simulink library "Soft_Starter_PLL"  (R2024a)
settings: Solver=VariableStepAuto  StartTime=0.0  StopTime=10.0  RelTol=1e-3
undefined symbols (not defined in the file or in its folder): D1, lagging, pulse
libraries: spsThyristorLib x6, spsThreePhaseParallelRLCBranchLib x3, spsThreePhaseBreakerLib x3, spsPLL3phLib x1, spsPulseGeneratorThyristor6PulseLib x1, simulink x1, spsThreePhaseVIMeasurementLib x1
settings Model: Creator=gshma  LastModifiedBy=gshma

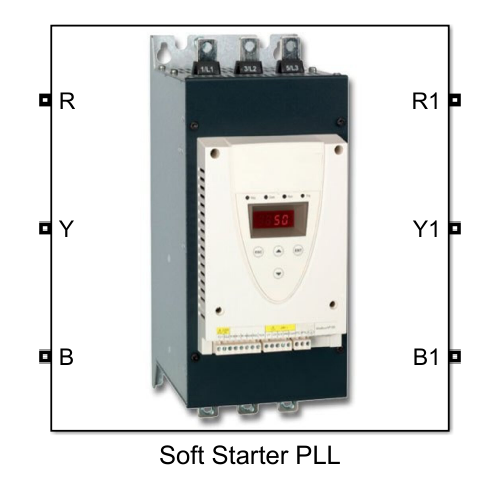
[thumbnail: Simulink's stored preview of the top-level diagram]
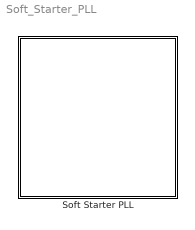
== system Soft_Starter_PLL ==
  Soft Starter PLL : Subsystem
      mask Display: image('schneider-altistart-01-soft-starter.jpeg');

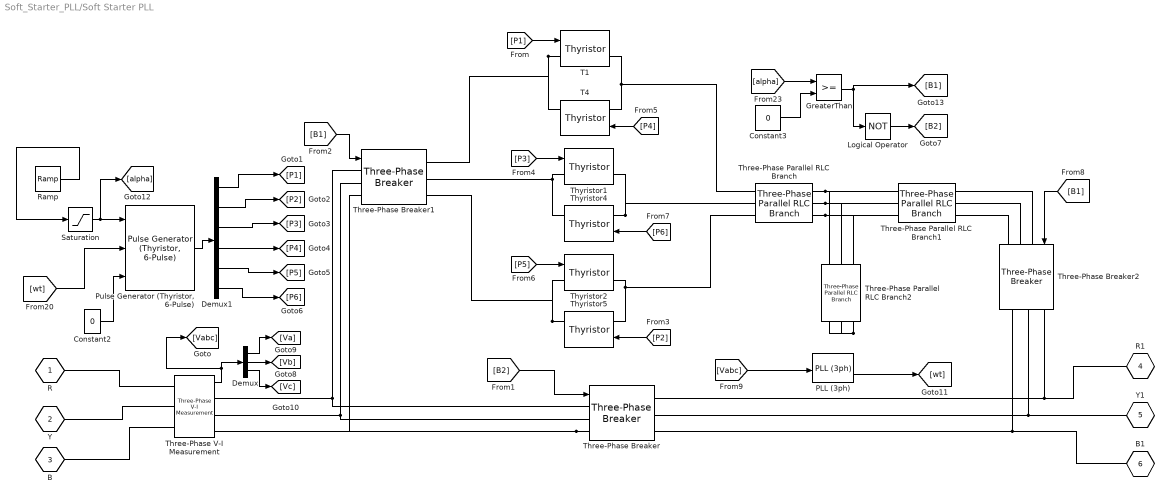
== system Soft_Starter_PLL/Soft Starter PLL ==
  Constant2 : Constant  Value=0
  Constant3 : Constant  Value=0
  Demux : Demux  Outputs=3
  Demux1 : Demux  Outputs=6
  GreaterThan : RelationalOperator  OutDataTypeStr=boolean  RndMeth=Simplest  InputSameDT=off
  Logical Operator : Logic  Operator=NOT  AllPortsSameDT=off  OutDataTypeStr=boolean
  PLL (3ph) : spsPLL3phLib/PLL (3ph)  Fmin=45  Par_Init=[0, 60]  ParK=[180, 3200, 1]  TcD=1e-4  MaxRateChangeFreq=12  FilterCutOffFreq=25  Ts=0  AGC=on
  "Pulse Generator (Thyristor, 6-Pulse)" : spsPulseGeneratorThyristor6PulseLib/Pulse Generator (Thyristor, 6-Pulse)  GenType=6-pulse  Delta=D1 (lagging)  pwidth=60  Double_Pulse=off  Ts=0
      settings: LibrarySourceBlock=|
      | sps_lib/Power Electronics/Power Electronics Control/Pulse Generator
      | (Thyristor, 6-Pulse)
  Ramp : simulink/Sources/Ramp  slope=-70  start=0.1  InitialOutput=90
  Saturation : Saturate  UpperLimit=90  LowerLimit=0
  T1 : spsThyristorLib/Thyristor  Ron=0.001  Lon=0  Vf=0.8  IC=0  Rs=500  Cs=250e-9  Measurements=on
  T4 : spsThyristorLib/Thyristor  Ron=0.001  Lon=0  Vf=0.8  IC=0  Rs=500  Cs=250e-9  Measurements=on
  Three-Phase Parallel RLC Branch : spsThreePhaseParallelRLCBranchLib/Three-Phase Parallel RLC Branch  LConnTagsString=A|B|C  RConnTagsString=A|B|C  BranchType=L  Resistance=1  Inductance=1e-3  Capacitance=1e-6  Measurements=None
  Three-Phase Parallel RLC Branch1 : spsThreePhaseParallelRLCBranchLib/Three-Phase Parallel RLC Branch  LConnTagsString=A|B|C  RConnTagsString=A|B|C  BranchType=L  Resistance=1  Inductance=2e-3  Capacitance=1e-6  Measurements=None
  Three-Phase Parallel RLC Branch2 : spsThreePhaseParallelRLCBranchLib/Three-Phase Parallel RLC Branch  LConnTagsString=A|B|C  RConnTagsString=A|B|C  BranchType=RC  Resistance=2  Inductance=38.25e-3  Capacitance=10e-6  Measurements=None
  Three-Phase V-I Measurement : spsThreePhaseVIMeasurementLib/Three-Phase V-I Measurement  VoltageMeasurement=phase-to-phase  SetLabelV=off  LabelV=Vabc  Vpu=off  VpuLL=off  CurrentMeasurement=no  SetLabelI=off  LabelI=Iabc  Ipu=off  Pbase=100e6  Vbase=500e3  OutputType=Complex  PhasorSimulation=off  PSBequivalent=0
  Three-Phase Breaker : spsThreePhaseBreakerLib/Three-Phase Breaker  InitialState=open  SwitchA=on  SwitchB=on  SwitchC=on  SwitchTimes="[1/60  5/60]"  External=on  BreakerResistance=0.01  SnubberResistance=1e6  SnubberCapacitance=inf  Measurements=None
  Three-Phase Breaker1 : spsThreePhaseBreakerLib/Three-Phase Breaker  InitialState=closed  SwitchA=on  SwitchB=on  SwitchC=on  SwitchTimes="[1/60  5/60]"  External=on  BreakerResistance=0.01  SnubberResistance=1e6  SnubberCapacitance=inf  Measurements=None
  Three-Phase Breaker2 : spsThreePhaseBreakerLib/Three-Phase Breaker  InitialState=closed  SwitchA=on  SwitchB=on  SwitchC=on  SwitchTimes="[1/60  5/60]"  External=on  BreakerResistance=0.01  SnubberResistance=1e6  SnubberCapacitance=inf  Measurements=None
  Thyristor{1..2,4..5} (4 alike) : spsThyristorLib/Thyristor  Ron=0.001  Lon=0  Vf=0.8  IC=0  Rs=500  Cs=250e-9  Measurements=on
  R : PMIOPort  Tag=simrfV2util1/Connection Port  Side=Left
  Y : PMIOPort  Tag=simrfV2util1/Connection Port  Port=2  Side=Left
  B : PMIOPort  Tag=simrfV2util1/Connection Port  Port=3  Side=Left
  R1 : PMIOPort  Tag=simrfV2util1/Connection Port  Port=4  Side=Right
  Y1 : PMIOPort  Tag=simrfV2util1/Connection Port  Port=5  Side=Right
  B1 : PMIOPort  Tag=simrfV2util1/Connection Port  Port=6  Side=Right
  wires:
  "Pulse Generator (Thyristor, 6-Pulse)"/1 -> Demux1/1
  Logical Operator/1 -> [B2]
  GreaterThan/1 -> [B1], Logical Operator/1
  Demux1/5 -> [P5]
  Constant3/1 -> GreaterThan/2
  Ramp/1 -> Saturation/1
  Three-Phase V-I Measurement/1 -> Demux/1, [Vabc]
  [alpha] -> GreaterThan/1
  Demux1/4 -> [P4]
  Demux/3 -> [Vc]
  Constant2/1 -> "Pulse Generator (Thyristor, 6-Pulse)"/3
  [P2] -> Thyristor5/1
  Demux1/3 -> [P3]
  Saturation/1 -> "Pulse Generator (Thyristor, 6-Pulse)"/1, [alpha]
  Demux1/1 -> [P1]
  [B1] -> Three-Phase Breaker1/1
  [P5] -> Thyristor2/1
  Demux1/2 -> [P2]
  [P6] -> Thyristor4/1
  [P1] -> T1/1
  Demux/2 -> [Vb]
  Demux/1 -> [Va]
  PLL (3ph)/2 -> [wt]
  [Vabc] -> PLL (3ph)/1
  [P3] -> Thyristor1/1
  [wt] -> "Pulse Generator (Thyristor, 6-Pulse)"/2
  Demux1/6 -> [P6]
  [B2] -> Three-Phase Breaker/1
  [P4] -> T4/1
  [B1] -> Three-Phase Breaker2/1
  connections:
  Three-Phase Breaker/LConn3 -- Three-Phase V-I Measurement/RConn3 -- Three-Phase Breaker1/LConn3
  Three-Phase Breaker1/RConn2 -- Thyristor4/RConn1 -- Thyristor1/LConn1
  Three-Phase Parallel RLC Branch2/LConn3 -- Three-Phase Parallel RLC Branch2/LConn1 -- Three-Phase Parallel RLC Branch2/LConn2
  Three-Phase Parallel RLC Branch/RConn3 -- Three-Phase Parallel RLC Branch1/LConn3 -- Three-Phase Parallel RLC Branch2/RConn3
  Thyristor5/RConn1 -- Thyristor2/LConn1 -- Three-Phase Breaker1/RConn3
  Three-Phase Parallel RLC Branch/LConn3 -- Thyristor5/LConn1 -- Thyristor2/RConn1
  Three-Phase Parallel RLC Branch/RConn1 -- Three-Phase Parallel RLC Branch1/LConn1 -- Three-Phase Parallel RLC Branch2/RConn1
  Three-Phase Breaker1/LConn1 -- Three-Phase Breaker/LConn1 -- Three-Phase V-I Measurement/RConn1
  Three-Phase Breaker1/LConn2 -- Three-Phase Breaker/LConn2 -- Three-Phase V-I Measurement/RConn2
  Three-Phase Parallel RLC Branch/RConn2 -- Three-Phase Parallel RLC Branch1/LConn2 -- Three-Phase Parallel RLC Branch2/RConn2
  Three-Phase Parallel RLC Branch/LConn1 -- T4/LConn1 -- T1/RConn1
  Thyristor4/LConn1 -- Thyristor1/RConn1 -- Three-Phase Parallel RLC Branch/LConn2
  Three-Phase Breaker/RConn3 -- Three-Phase Breaker2/RConn3 -- B1/RConn1
  Three-Phase Breaker/RConn2 -- Y1/RConn1 -- Three-Phase Breaker2/RConn2
  Three-Phase Breaker/RConn1 -- Three-Phase Breaker2/RConn1 -- R1/RConn1
  T1/LConn1 -- T4/RConn1 -- Three-Phase Breaker1/RConn1
  B/RConn1 -- Three-Phase V-I Measurement/LConn3
  Y/RConn1 -- Three-Phase V-I Measurement/LConn2
  R/RConn1 -- Three-Phase V-I Measurement/LConn1
  Three-Phase Breaker2/LConn1 -- Three-Phase Parallel RLC Branch1/RConn1
  Three-Phase Breaker2/LConn2 -- Three-Phase Parallel RLC Branch1/RConn2
  Three-Phase Breaker2/LConn3 -- Three-Phase Parallel RLC Branch1/RConn3
